simulink model "chap6_11input"  (R2019a)
settings: Solver=ode45  StartTime=0.0  StopTime=10.0  RelTol=1e-3
settings Model: Creator=smilingfrog  LastModifiedBy=smilingfrog

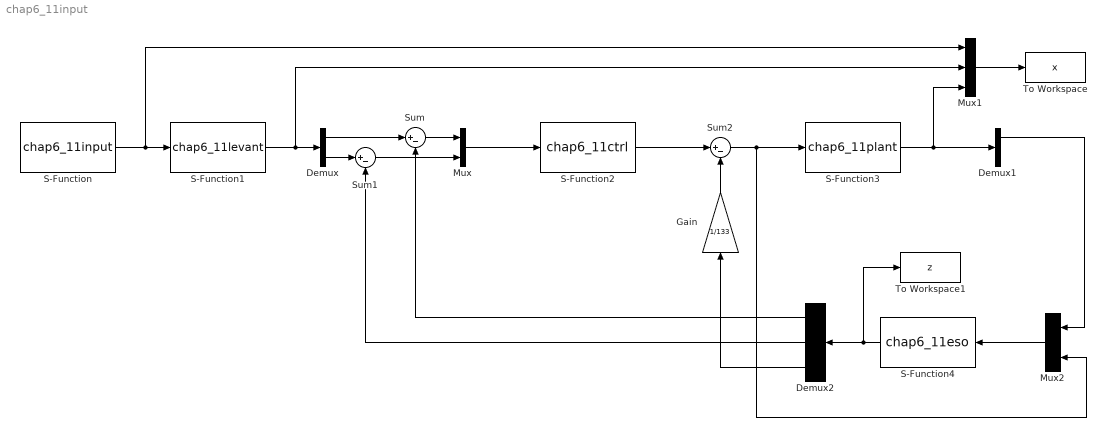
== system chap6_11input ==
  Demux : Demux  Outputs=2
  Demux1 : Demux  Outputs=3
  Demux2 : Demux  Outputs=3
  Gain : Gain  Gain=1/133
  Mux : Mux  Inputs=2
  Mux1 : Mux  Inputs=3
  Mux2 : Mux  Inputs=2
  S-Function : S-Function  FunctionName=chap6_11input  SFunctionDeploymentMode=off  EnableBusSupport=off
  S-Function1 : S-Function  FunctionName=chap6_11levant  SFunctionDeploymentMode=off  EnableBusSupport=off
  S-Function2 : S-Function  FunctionName=chap6_11ctrl  SFunctionDeploymentMode=off  EnableBusSupport=off
  S-Function3 : S-Function  FunctionName=chap6_11plant  SFunctionDeploymentMode=off  EnableBusSupport=off
  S-Function4 : S-Function  FunctionName=chap6_11eso  SFunctionDeploymentMode=off  EnableBusSupport=off
  Sum : Sum  Inputs=|+-
  Sum1 : Sum  Inputs=|+-
  Sum2 : Sum  Inputs=|+-
  To Workspace : ToWorkspace  VariableName=x  SampleTime=-1
  To Workspace1 : ToWorkspace  VariableName=z  SampleTime=-1
  wires:
  S-Function/1 -> Mux1/1, S-Function1/1
  S-Function1/1 -> Mux1/2, Demux/1
  Demux/1 -> Sum/1
  Sum/1 -> Mux/1
  Demux/2 -> Sum1/1
  Sum1/1 -> Mux/2
  Mux/1 -> S-Function2/1
  S-Function2/1 -> Sum2/1
  Gain/1 -> Sum2/2
  S-Function3/1 -> Demux1/1, Mux1/3
  Mux1/1 -> To Workspace/1
  Demux1/1 -> Mux2/1
  Mux2/1 -> S-Function4/1
  S-Function4/1 -> To Workspace1/1, Demux2/1
  Sum2/1 -> Mux2/2, S-Function3/1
  Demux2/3 -> Gain/1
  Demux2/1 -> Sum/2
  Demux2/2 -> Sum1/2
